simulink model "MDLL_rab_1"  (Simulink 7.4)
settings: Solver=ode45  StartTime=0.0  StopTime=10e-4  FixedStep=1e-9  MaxStep=1e-8  RelTol=1e-3
libraries: simulink x4, simulink_extras x2
settings Model: Creator=Dick Benson  LastModifiedBy=Dick
settings SolverCC: ZeroCrossControl=EnableAll

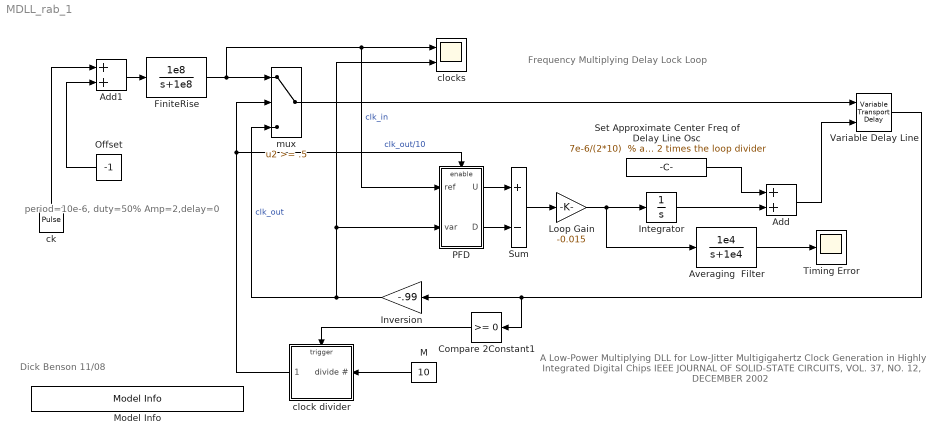
== system MDLL_rab_1 ==
  note: period=10e-6,
      | duty=50%
      | Amp=2,delay=0
  note: Frequency Multiplying Delay Lock Loop
  note: A Low-Power Multiplying DLL for Low-Jitter
      | Multigigahertz Clock Generation in Highly
      | Integrated Digital Chips
      | IEEE JOURNAL OF SOLID-STATE CIRCUITS, VOL. 37, NO. 12, DECEMBER 2002
  note: Dick Benson
      | 11/08
  Add : Sum  OutDataType=sfix(16)  OutScaling=2^-10
  Add1 : Sum  OutDataType=sfix(16)  OutScaling=2^-10
  Averaging  Filter : TransferFcn  Numerator=[1e4]  Denominator=[1 1e4]
  Compare 2Constant1 : simulink/Logic and Bit Operations/Compare To Constant  SystemSampleTime=-1  relop=>=  const=0  LogicOutDataTypeMode=boolean  ZeroCross=off
  FiniteRise : TransferFcn  Numerator=[1e8]  Denominator=[1 1e8]
  Integrator : Integrator
  Inversion : Gain  Gain=-.99  ParameterDataType=sfix(16)  ParameterScaling=2^0  OutDataType=sfix(16)  OutScaling=2^0
  Loop Gain : Gain  Gain=-0.015  ParameterDataType=sfix(16)  ParameterScaling=2^0  OutDataType=sfix(16)  OutScaling=2^0
  M : Constant  Value=10  OutDataType=sfix(16)  OutScaling=2^0
  Model Info : simulink/Model-Wide Utilities/Model Info  SystemSampleTime=-1  InitialBlockCM=None  BlockCM=None  Frame=on  DisplayStringWithTags=Copywrite 2008-2010 The MathWorks, Inc.  HorizontalTextAlignment=Center  LeftAlignmentValue=0.5  SourceBlockDiagram=MDLL_rab_1  TagMaxNumber=20
  Offset : Constant  Value=-1  OutDataType=sfix(16)  OutScaling=2^0
  PFD : Subsystem
  Set Approximate Center Freq of Delay Line Osc : Constant  Value="7e-6/(2*10)  % apporximate target clock period divided by 2 times the loop divider"  OutDataType=sfix(16)  OutScaling=2^0
  Sum : Sum  Inputs=+-  SaturateOnIntegerOverflow=on  InputSameDT=on  OutDataTypeStr=Inherit: Same as first input
  Timing Error : Scope
      settings: TimeRange=0.001  YMin=-0.001  YMax=0.001  MaxDataPoints=150000
  Variable Delay Line : VariableTransportDelay  MaximumDelay=64e-6  InitialOutput=1  MaximumPoints=8192
  ck : DiscretePulseGenerator  PulseType=Time based  Amplitude=2  Period=10e-6  PulseWidth=50  PhaseDelay=0  SampleTime=1
  clock divider : Subsystem  TreatAsAtomicUnit=on
  clocks : Scope  NumInputPorts=2
      settings: TimeRange=2e-005  YMin=-1.2~-1.2  YMax=1.2~1.2  MaxDataPoints=50000
  mux : Switch  Threshold=.5  SaturateOnIntegerOverflow=on  InputSameDT=on
  wires:
  PFD/1(U) -> Sum/1
  PFD/2(D) -> Sum/2
  Sum/1 -> Loop Gain/1
  Integrator/1 -> Add/2
  Add/1 -> Variable Delay Line/2
  mux/1 -> Variable Delay Line/1
  clock divider/1(" ") -> mux/2, PFD/Enable  "clk_out/10"
  M/1 -> clock divider/1("divide # ")
  Variable Delay Line/1 -> Inversion/1, Compare 2Constant1/1
  Inversion/1 -> mux/3, PFD/2(var), clocks/2  "clk_out"
  Set Approximate Center Freq of Delay Line Osc/1 -> Add/1
  FiniteRise/1 -> mux/1, clocks/1, PFD/1(ref)  "clk_in"
  Add1/1 -> FiniteRise/1
  Offset/1 -> Add1/2
  Averaging  Filter/1 -> Timing Error/1
  Loop Gain/1 -> Integrator/1, Averaging  Filter/1
  ck/1 -> Add1/1
  Compare 2Constant1/1 -> clock divider/Trigger

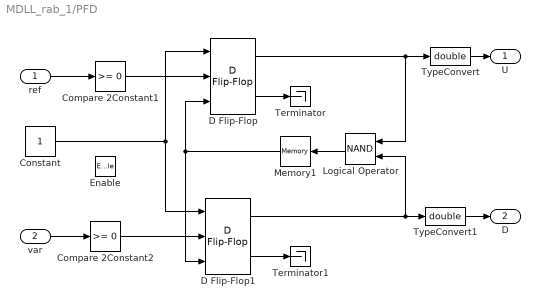
== system MDLL_rab_1/PFD ==
  ref : Inport  OutDataType=sfix(16)  OutScaling=2^0
  var : Inport  Port=2  OutDataType=sfix(16)  OutScaling=2^0
  Enable : EnablePort
  Compare 2Constant1 : simulink/Logic and Bit Operations/Compare To Constant  SystemSampleTime=-1  relop=>=  const=0  LogicOutDataTypeMode=boolean  ZeroCross=off
  Compare 2Constant2 : simulink/Logic and Bit Operations/Compare To Constant  SystemSampleTime=-1  relop=>=  const=0  LogicOutDataTypeMode=boolean  ZeroCross=off
  Constant : Constant  OutDataTypeMode=boolean  OutDataType=sfix(16)  OutScaling=2^0  OutDataTypeStr=boolean
  D Flip-Flop : simulink_extras/Flip Flops/D Flip-Flop  SystemSampleTime=-1
  D Flip-Flop1 : simulink_extras/Flip Flops/D Flip-Flop  SystemSampleTime=-1
  Logical Operator : Logic  Operator=NAND
  Memory1 : Memory
  Terminator : Terminator
  Terminator1 : Terminator
  TypeConvert : DataTypeConversion  OutDataTypeMode=double  OutDataType=sfix(16)  OutScaling=2^0  OutDataTypeStr=double  RndMeth=Nearest
  TypeConvert1 : DataTypeConversion  OutDataTypeMode=double  OutDataType=sfix(16)  OutScaling=2^0  OutDataTypeStr=double  RndMeth=Nearest
  U : Outport  OutDataType=sfix(16)  OutScaling=2^0  OutputWhenDisabled=reset  InitialOutput=0
  D : Outport  Port=2  OutDataType=sfix(16)  OutScaling=2^0  OutputWhenDisabled=reset  InitialOutput=0
  wires:
  var/1 -> Compare 2Constant2/1
  D Flip-Flop/2 -> Terminator/1
  D Flip-Flop1/2 -> Terminator1/1
  ref/1 -> Compare 2Constant1/1
  Constant/1 -> D Flip-Flop/1, D Flip-Flop1/1
  Memory1/1 -> D Flip-Flop/3, D Flip-Flop1/3
  D Flip-Flop/1 -> Logical Operator/1, TypeConvert/1
  D Flip-Flop1/1 -> Logical Operator/2, TypeConvert1/1
  Logical Operator/1 -> Memory1/1
  TypeConvert/1 -> U/1
  TypeConvert1/1 -> D/1
  Compare 2Constant2/1 -> D Flip-Flop1/2
  Compare 2Constant1/1 -> D Flip-Flop/2

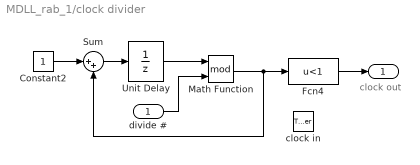
== system MDLL_rab_1/clock divider ==
  note: clock out
  "divide # " : Inport  OutDataType=sfix(16)  OutScaling=2^0
  clock in : TriggerPort
  Constant2 : Constant  OutDataType=sfix(16)  OutScaling=2^0
  Fcn4 : Fcn  Expr=u<1
  Math Function : Math  Operator=mod  OutDataType=sfix(16)  OutScaling=2^0  SaturateOnIntegerOverflow=on
  Sum : Sum  Inputs=|++  OutDataType=sfix(16)  OutScaling=2^0  SaturateOnIntegerOverflow=on  InputSameDT=on  OutDataTypeStr=Inherit: Same as first input
  Unit Delay : UnitDelay  SampleTime=-1
  " " : Outport  OutDataType=sfix(16)  OutScaling=2^0
  wires:
  "divide # "/1 -> Math Function/2
  Fcn4/1 -> " "/1
  Math Function/1 -> Fcn4/1, Sum/2
  Unit Delay/1 -> Math Function/1
  Constant2/1 -> Sum/1
  Sum/1 -> Unit Delay/1
